simulink model "OCTModel"  (R2018b)
settings: Solver=ode23s  StartTime=0.0  StopTime=duration_s  FixedStep=0.1  MaxStep=0.1*sqrt(lengthScaleFactor)  RelTol=1e-3  AbsTol=1e-3
libraries: animation_cl x1, environment_cl x1, flightController_cl x1, gndStnController_cl x1, hiLvlController_cl x1, plant_cl x1
PreSaveFcn:
  | % Callback to reset the view so that the
  | % the next person to open isn't totally lost.
  | hilite_system('OCTModel/plant');
  | hilite_system('OCTModel/plant','none');
  | set_param(gcs,'Zoomfactor','fit to view')
settings Model: SimulationMode=accelerator  ExtModeTrigDuration=100  Creator=mcobb  LastModifiedBy=jldanie5
settings SolverCC: SolverResetMethod=Robust
settings DataIOCC: SaveOutput=off  DSMLogging=off  StateSaveName=tmp_raccel_xout
settings OptimizationCC: EfficientMapNaN2IntZero=off
settings DebuggingCC: SignalRangeChecking=error  ArtificialAlgebraicLoopMsg=none
settings HardwareCC: TargetBitPerPointer=64  TargetBitPerSizeT=64  TargetBitPerPtrDiffT=64  TargetLongLongMode=on  TargetIntDivRoundTo=Zero  TargetEndianess=LittleEndian  TargetWordSize=64  TargetHWDeviceType=MATLAB Host  ProdEqTarget=off
settings RTWCC: SystemTargetFile=raccel.tlc  TemplateMakefile=raccel_default_tmf  RTWVerbose=off  RTWUseSimCustomCode=on
settings CodeAppCC: GenerateComments=off  MaxIdLength=128  MangleLength=10
settings RaccelTargetCC: GeneratePreprocessorConditionals=Use local settings  MultiInstanceERTCode=off  PreserveStateflowLocalDataDimensions=off  ENABLE_SLEXEC_SSBRIDGE=1  RTWCAPIParams=on

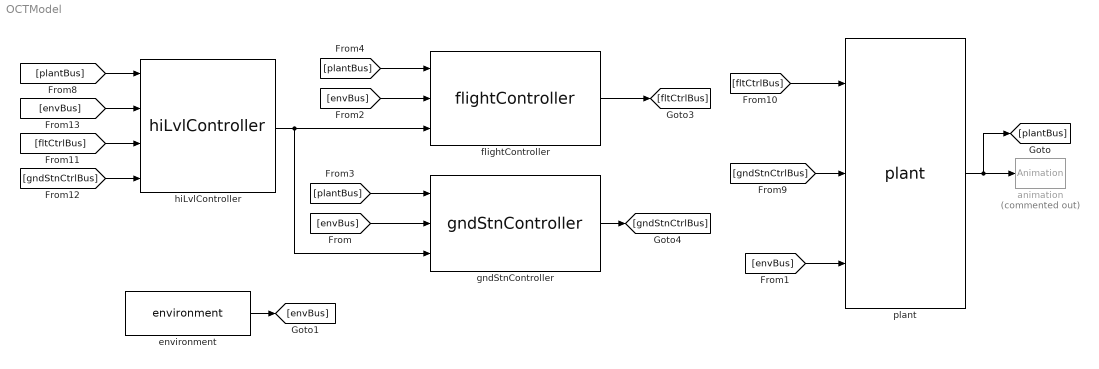
== system OCTModel ==
  animation : animation_cl/Animation  Commented=on  animSampleTime=0.1  scaleFactor=scaleFactor  elevation=45  radius=500  vidLogEnbl=off  vidDims=[240 480]*2
  environment : environment_cl/environment  SystemSampleTime=-1
  flightController : flightController_cl/flightController  SystemSampleTime=-1
      link override pathFollowingController/Selector: InputPortWidth=1000
  gndStnController : gndStnController_cl/gndStnController  SystemSampleTime=-1
      link override anchorTetherCtrl: ctrl=gndCtrl
  hiLvlController : hiLvlController_cl/hiLvlController  SystemSampleTime=-1
  plant : plant_cl/plant  SystemSampleTime=-1  VariantControl=VSS_plant_modularPlant
      link override groundStation/groundStation001: anchWnchStruct=anchWnch.struct('OCT.winch')  numNodes=gndStn.anchThrs.numNodes.Value  e=env
      link override vehicle/vehicle000/fluidDynamicSurface: aeroStruct=vcl.struct('OCT.aeroSurf')
      link override vehicle/vehicle000/fuselage/Constant6: Value=fus.sideDragCoeff.Value
      link override vehicle/vehicle000/sixDoFDynamics: M_added=vhcl.addedMass.Value  J_added=vhcl.addedInertia.Value
  wires:
  plant/1 -> [plantBus], animation/1
  environment/1 -> [envBus]
  [envBus] -> gndStnController/2
  [envBus] -> plant/3
  [envBus] -> flightController/2
  [plantBus] -> gndStnController/1
  [plantBus] -> flightController/1
  [plantBus] -> hiLvlController/1
  flightController/1 -> [fltCtrlBus]
  gndStnController/1 -> [gndStnCtrlBus]
  [gndStnCtrlBus] -> plant/2
  [fltCtrlBus] -> plant/1
  [envBus] -> hiLvlController/2
  [fltCtrlBus] -> hiLvlController/3
  [gndStnCtrlBus] -> hiLvlController/4
  hiLvlController/1 -> gndStnController/3, flightController/3
